simulink model "chap2_1sim"  (Simulink 5.0)
settings: Solver=ode45  StartTime=0.0  StopTime=10  FixedStep=0.001  RelTol=1e-3
settings Model: LastModifiedBy=Administrator  ExtModeTrigMode=oneshot  ExtModeArmWhenConnect=off  LimitDataPoints=off  BooleanDataType=off

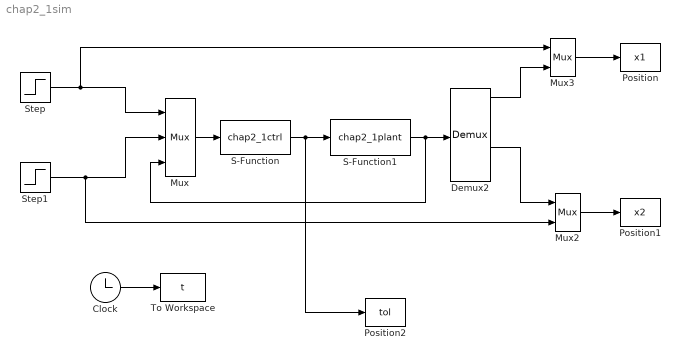
== system chap2_1sim ==
  Clock : Clock
      settings: Decimation=10
  Demux2 : Demux
  Mux : Mux  Inputs=3
  Mux2 : Mux  Inputs=2
  Mux3 : Mux  Inputs=2
  Position : ToWorkspace  VariableName=x1  SampleTime=-1  SaveFormat=Array
  Position1 : ToWorkspace  VariableName=x2  SampleTime=-1  SaveFormat=Array
  Position2 : ToWorkspace  VariableName=tol  SampleTime=-1  SaveFormat=Array
  S-Function : S-Function  FunctionName=chap2_1ctrl
  S-Function1 : S-Function  FunctionName=chap2_1plant
  Step : Step  Time=0  SampleTime=0
  Step1 : Step  Time=0  SampleTime=0
  To Workspace : ToWorkspace  VariableName=t  SampleTime=-1  SaveFormat=Array
  wires:
  Mux/1 -> S-Function/1
  Mux2/1 -> Position1/1
  Step/1 -> Mux/1, Mux3/1
  Mux3/1 -> Position/1
  S-Function/1 -> S-Function1/1, Position2/1
  Step1/1 -> Mux/2, Mux2/2
  Demux2/1 -> Mux3/2
  S-Function1/1 -> Demux2/1, Mux/3
  Demux2/3 -> Mux2/1
  Clock/1 -> To Workspace/1
